simulink model "lab4p2c"  (R2023b)
settings: Solver=ode23tb  StartTime=0.0  StopTime=Tmdl  FixedStep=To/100  MaxStep=To/100  RelTol=1e-3
undefined symbols (not defined in the file or in its folder): an, dsc, T, To
settings Model: Creator=deniskirbaba  LastModifiedBy=Max

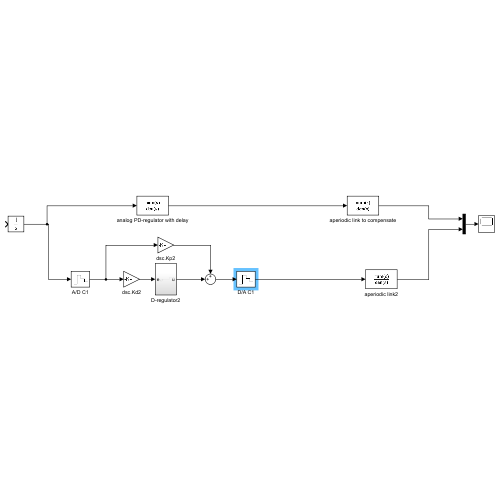
[thumbnail: Simulink's stored preview of the top-level diagram]
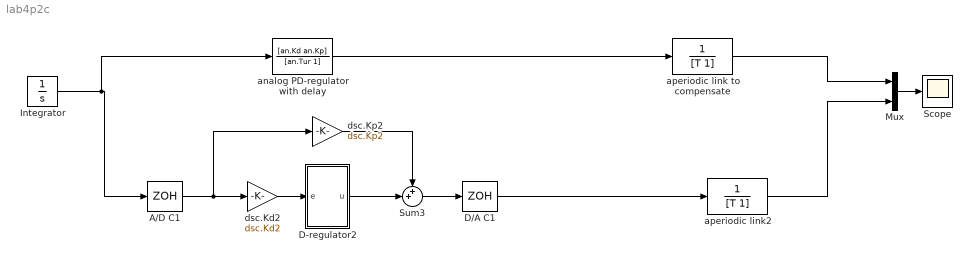
== system lab4p2c ==
  A/D C1 : ZeroOrderHold  SampleTime=To
  D-regulator2 : Subsystem
  D/A C1 : ZeroOrderHold  SampleTime=To
  Integrator : Integrator  InitialCondition=1
  Mux : Mux  Inputs=2
  Scope : Scope
  Sum3 : Sum  Inputs=++|
  analog PD-regulator with delay : TransferFcn  Numerator=[an.Kd an.Kp]  Denominator=[an.Tur 1]
  aperiodic link to compensate : TransferFcn  Denominator=[T 1]
  aperiodic link2 : TransferFcn  Denominator=[T 1]
  dsc.Kd2 : Gain  Gain=dsc.Kd2
  dsc.Kp2 : Gain  Gain=dsc.Kp2
  wires:
  Mux/1 -> Scope/1
  aperiodic link to compensate/1 -> Mux/1
  aperiodic link2/1 -> Mux/2
  D/A C1/1 -> aperiodic link2/1
  dsc.Kp2/1 -> Sum3/1
  A/D C1/1 -> dsc.Kp2/1, dsc.Kd2/1
  Sum3/1 -> D/A C1/1
  dsc.Kd2/1 -> D-regulator2/1(e)
  D-regulator2/1(u) -> Sum3/2
  Integrator/1 -> analog PD-regulator with delay/1, A/D C1/1
  analog PD-regulator with delay/1 -> aperiodic link to compensate/1

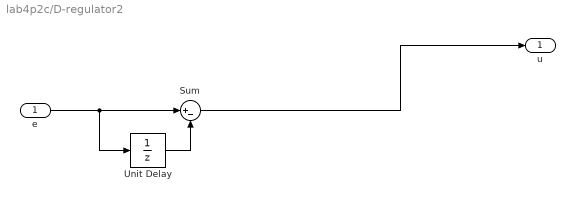
== system lab4p2c/D-regulator2 ==
  e : Inport
  Sum : Sum  Inputs=|+-
  Unit Delay : UnitDelay  SampleTime=To  HasFrameUpgradeWarning=on
  u : Outport
  wires:
  Sum/1 -> u/1
  Unit Delay/1 -> Sum/2
  e/1 -> Unit Delay/1, Sum/1
